simulink library "HEV_Battery_Lib"  (R2019b)
settings: Solver=ode45  StartTime=0.0  StopTime=10.0  RelTol=1e-3  EnableMultiTasking=on
undefined symbols (not defined in the file): HEV_Param, Hydride, Kt_Temps, Metal, Nickel
libraries: fl_lib x55, nesl_utility x30, LeadAcidBattery_lib x12, $bdroot x9, fl_ps_legacy_lib x9, ee_lib x3, powerlib x3, Capacitors_lib x1, electricdrivelib x1
(part 2 of 2)

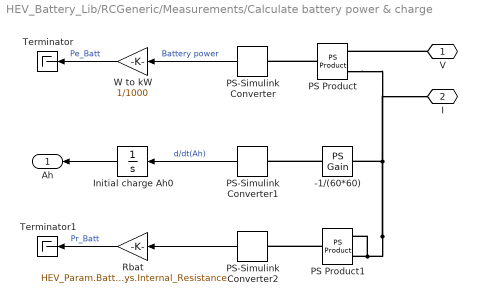
== system HEV_Battery_Lib/RCGeneric/Measurements/Calculate battery power & charge ==
  -1/(60*60) : fl_ps_legacy_lib/Legacy Physical Signals/Functions/PS Gain  gain=-1/(60*60)
      settings: SourceProductName=Simscape
  Initial charge Ah0 : Integrator  InitialCondition=HEV_Param.Battery_Sys.Maximum_Capacity
  PS Product : fl_ps_legacy_lib/Legacy Physical Signals/Functions/PS Product
      settings: SourceProductName=Simscape  SourceProductBaseCode=SS
  PS Product1 : fl_ps_legacy_lib/Legacy Physical Signals/Functions/PS Product
      settings: SourceProductName=Simscape  SourceProductBaseCode=SS
  PS-Simulink Converter : nesl_utility/PS-Simulink Converter  PhysicalDomain=network_engine_domain  SubClassName=ps_output  LeftPortType=input  RightPortType=output  PseudoPeriodic=off  Frequencies=[]  Unit=W  AffineConversion=off
  PS-Simulink Converter1 : nesl_utility/PS-Simulink Converter  PhysicalDomain=network_engine_domain  SubClassName=ps_output  LeftPortType=input  RightPortType=output  PseudoPeriodic=off  Frequencies=[]  Unit=1  AffineConversion=off
  PS-Simulink Converter2 : nesl_utility/PS-Simulink Converter  PhysicalDomain=network_engine_domain  SubClassName=ps_output  LeftPortType=input  RightPortType=output  PseudoPeriodic=off  Frequencies=[]  Unit=1  AffineConversion=off
  Rbat : Gain  Gain=HEV_Param.Battery_Sys.Internal_Resistance
  Terminator : Terminator
  Terminator1 : Terminator
  W to kW : Gain  Gain=1/1000
  V : PMIOPort  Side=Left
  I : PMIOPort  Port=2  Side=Left
  Ah : Outport
  wires:
  Rbat/1 -> Terminator1/1  "Pr_Batt"
  PS-Simulink Converter2/1 -> Rbat/1
  Initial charge Ah0/1 -> Ah/1
  PS-Simulink Converter1/1 -> Initial charge Ah0/1  "d/dt(Ah)"
  W to kW/1 -> Terminator/1  "Pe_Batt"
  PS-Simulink Converter/1 -> W to kW/1  "Battery power"
  connections:
  PS Product1/RConn1 -- PS-Simulink Converter2/LConn1
  -1/(60*60)/RConn1 -- PS-Simulink Converter1/LConn1
  PS Product1/LConn2 -- PS Product1/LConn1 -- -1/(60*60)/LConn1 -- I/RConn1 -- PS Product/LConn2
  V/RConn1 -- PS Product/LConn1
  PS Product/RConn1 -- PS-Simulink Converter/LConn1
